simulink model "ysw13_4"  (Simulink 8.3)
settings: Solver=ode4  StartTime=0.0  StopTime=1.0  RelTol=1e-3
undefined symbols (not defined in the file or in its folder): ysw13_4ctrl
settings Model: Creator=Administrator  LastModifiedBy=Administrator  ExtModeTrigMode=oneshot  ExtModeArmWhenConnect=off
settings DataIOCC: Decimation=100  LimitDataPoints=off  SaveOutput=off  SaveTime=off
settings OptimizationCC: BlockReduction=off  BooleanDataType=off  InitFltsAndDblsToZero=on
settings DebuggingCC: SaveWithParameterizedLinksMsg=none  SignalResolutionControl=TryResolveAllWithWarning  SolverPrmCheckMsg=none  MultiTaskDSMMsg=warning  MultiTaskCondExecSysMsg=none  FcnCallInpInsideContextMsg=UseLocalSettings  StateNameClashWarn=none
settings HardwareCC: TargetUnknown=on
settings RTWCC: IncludeERTFirstTime=on
settings GRTTargetCC: TargetFcnLib=ansi_tfl_tmw.mat

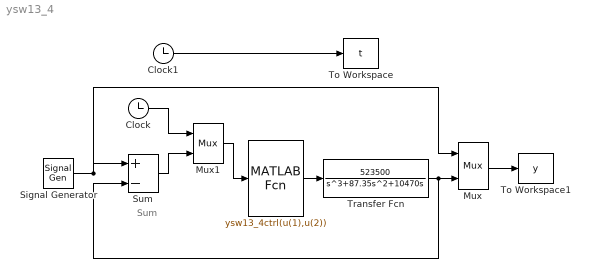
== system ysw13_4 ==
  note: Sum
  "    " : MATLABFcn  MATLABFcn=ysw13_4ctrl(u(1),u(2))
  Clock : Clock
  Clock1 : Clock
  Mux : Mux  Inputs=2
  Mux1 : Mux  Inputs=2
  Signal Generator : SignalGenerator  Amplitude=0.05
  Sum : Sum  Inputs=|+-  SaturateOnIntegerOverflow=on  InputSameDT=on  OutDataTypeStr=Inherit: Same as first input
  To Workspace : ToWorkspace  VariableName=t  SampleTime=-1
  To Workspace1 : ToWorkspace  VariableName=y  SampleTime=-1
  Transfer Fcn : TransferFcn  Numerator=[523500]  Denominator=[1 87.35 10470 0]
  wires:
  Mux/1 -> To Workspace1/1
  Transfer Fcn/1 -> Sum/2, Mux/2
  Signal Generator/1 -> Sum/1, Mux/1
  Clock/1 -> Mux1/1
  Sum/1 -> Mux1/2
  Mux1/1 -> "    "/1
  "    "/1 -> Transfer Fcn/1
  Clock1/1 -> To Workspace/1
